simulink model "HDVSim_Dual_Fuel_Hybrid_Truck"  (R2018b)
settings: Solver=ode3  StartTime=0.0  StopTime=inf  FixedStep=sample_time  MaxStep=0.1  RelTol=1e-3  EnableMultiTasking=on
model workspace (MAT data in the model file):
  Bat.Useable_capacity = 30.52398723
  Bat.Useable_range = 0.302889592
  Bat.Type = 2
  Bat.SOC_start = 1
  Bat.Voltage = 800
  Bat.Charge_cycles = 14203.5582315
  Bat.Efficiency_power_electronics = 0.95
  Electric_Truck = 0
  Fueltype = 11
  Hybrid_Truck = 1
  IZ12 = 3600
  SOC_T_EM_completely_available = 0.089152566
  SOC_addition = 0.262901104
  SOC_target = 0
  Sailing_without_drag_torque = 1
  TCO = TCO
  TCO.Ratio_Trailer_Truck = [1 1]
  TCO.Price_increase_repurchase = [3.5 3.5]
  TCO.Daily_working_time = 8
  TCO.Other_works_day = 0.5
  TCO.Gross_hourly_wage_driver = 13
  TCO.Operating_days_year = 240
  TCO.Annual_gross_wage_driver = 24960
  TCO.Personnel_factor = 1.3
  TCO.Annual_gross_wage_truck = 32448
  TCO.Social_costs_percent = 25.75
  TCO.Social_costs_EUR = 8355
  TCO.Back_up_driver = 0
  TCO.Fees_day = 12
  TCO.Fees_year = 2880
  TCO.Driver_costs_other = 0
  TCO.Driving_personnel_costs_total = 43683
  TCO.Diesel_price = 0.95
  TCO.Diesel_price_external = 1
  TCO.Adblue_price = 0.68
  TCO.CNG_price = 0.88
  TCO.LNG_price = 0.81
  TCO.Electricity_price = 0.12
  TCO.Hydrogen_price = 9
  TCO.Interest_current_asset = 8.4
  TCO.Interest_fixed_asset = 8.4
  TCO.Administrative_costs = 10.7
  TCO.Driving_distance = 0
  TCO.Ratio_toll_route = 75
  TCO.Loading_time_combination = 0.25
  TCO.Unloading_time_combination = 0.25
  TCO.Ratio_empty_trips = 0
  TCO.Operating_life = [6 12]
  TCO.Tire_mileage = [140000 170000]
  TCO.Ratio_inhouse_tanking_diesel = 75
  TCO.Lubricant_consumption = 1
  TCO.Adblue_consumption = 4
  TCO.Afa_time_dependent = [100 100]
  TCO.Afa_power_dependent = [0 0]
  TCO.Current_asset = [6000 1400]
  TCO.Insurance_vehicle = [0 0]
  TCO.Insurance_transport = 1000
  TCO.Communication = 600
  TCO.Repair_maintenance_care = [0.13 0.025]
  TCO.Current_assets_interest_bearing = 622
  TCO.Results = table
  TCO.Results.data = {{[]; []; []; []; []; []; []; []; []; []; []; []; []; []; []; []; []; []; []; []; []; []; []}, {[]; []; []; []; []; []; []; []; []; []; []; []; []; []; []; []; []; []; []; []; []; []; []}, {[]; []; []; []; []; []; []; []; []; []; []; []; []; []; []; []; []; []; []; []; []; []; []}, {'#cccccc'; '#9DFF00'; '#CEFF00'; '#FFFF00'; '#FFDF00'; '#FFB900'; '#FF9200'; '#FF5D00'; '#FF7F7F'; '#FF2900'; '#cccccc'; '#00FF85'; '#00FFC6'; '#00FFF2'; '#00FFFF'; '#00DBFF'; '#00B3FF'; '#0088FF'; '#cccccc'; '#B100FF'; '#FF00FF'; '#FF00C0'; '#FF0070'}, [0; 1; 1; 1; 1; 1; 1; 0; 1; 0; 0; 1; 1; 1; 1; 1; 1; 0; 0; 0; 1; 1; 0]}
  TCO.Results.ndims = 2
  TCO.Results.nrows = 23
  TCO.Results.rownames = {'Time_dependent_vehicle_costs'; 'Amortisation_time_dependent'; 'Current_assets_interest_bearing'; 'Fixed_assets_interest_bearing'; 'Taxes'; 'Insurance'; 'Communication'; 'Sum_vehicle_costs'; 'Driving_personnel_costs_total'; 'Sum_fix_costs'; 'Performance_related_vehicle_costs'; 'Amortisation_performance_related'; 'Fuel_costs'; 'Adblue_costs'; 'Repair_costs'; 'Lubricant_costs'; 'Tire_costs'; 'Sum_variable_costs'; 'Sum_costs'; 'Sum_fix_variable_costs'; 'Overhead_costs'; 'Toll_costs'; 'Total_costs'}
  TCO.Results.nvars = 5
  TCO.Results.varnames = {'Euro_Year', 'Euro_km', 'Percent', 'Cellcolor', 'Diagramm'}
  TCO.Results.props.CustomProps = struct()
  TCO.Results.props.VariableCustomProps = struct()
  TCO.Results.props.versionSavedFrom = 3
  TCO.Results.props.minCompatibleVersion = 1
  TCO.Results.props.incompatibilityMsg = ''
  TCO.Results.props.VersionSavedFrom = 3
  TCO.Results.props.Description = ''
  TCO.Results.props.DimensionNames = {'Row', 'Variables'}
  TCO.Results.props.UserData = []
  TCO.Results.props.VariableDescriptions = {}
  TCO.Results.props.VariableUnits = {}
  TCO.Results.props.VariableContinuity = {}
  TCO_Trailer = 1
  T_distance_LPS_down = 500
  T_distance_LPS_up = 434.9496342
  VSim.Display = 3
  VSim.Opt = 0
  Vehicle = 'LNGDieselHybrid'
  WPT.Voltage = 0
  WPT.P_max = 200
  WPT.expansion = 0.3
  WPT.eta = 0.92
  WPT.SOC_target = 0.8
  WPT.SOC_electric_only = 0.3
  acquisitionCosts = acquisitionCosts
  acquisitionCosts.KA_ZM = 141266.812415
  acquisitionCosts.KG = 5816.60979338
  acquisitionCosts.Getr_m = 249.375588545
  acquisitionCosts.KMot = 21229.1233715
  acquisitionCosts.Motor_Mmax = 1810.391452
  acquisitionCosts.Motor_m = 882.849968657
  acquisitionCosts.KH = 16865.1016034
  acquisitionCosts.Hybrid = 1
  acquisitionCosts.Bat = 14389.2541556
  acquisitionCosts.Bat_type = 2
  acquisitionCosts.Bat_m = 500.750076074
  acquisitionCosts.Bat_kWh = 80.6207622479
  acquisitionCosts.Ratio_BEV2PHEV = 1
  acquisitionCosts.EM = 1329.27467614
  acquisitionCosts.EM_Type = 1
  acquisitionCosts.EM_P_max = 103.365060353
  acquisitionCosts.LE = 465.142771589
  acquisitionCosts.FC = 0
  acquisitionCosts.P_FC = 0
  acquisitionCosts.KA = 6181
  acquisitionCosts.v_diesel = 300
  acquisitionCosts.v_cng = 0
  acquisitionCosts.v_lng = 300
  acquisitionCosts.m_h2 = 0
  acquisitionCosts.KT = 4182.16
  acquisitionCosts.KTD = 292.81
  acquisitionCosts.KTCNG = 0
  acquisitionCosts.KTLNG = 3889.35
  acquisitionCosts.KTFC = 0
  addition_for_critical_slope = 0.030662181
  ambient.gravity = 9.80665
  ambient.air_density = 1.1883
  ambient.friction_coeff = 0.8
  auxiliary_consumers.onBattery = 0
  auxiliary_consumers.power = 3500
  critical_altitude_difference = 39.0505026
  cycle.distance = [0 1 2 3 4 5 6 7 8 9 10 11 ... (3001 elements, 3001x1)]
  cycle.speed = [0 24.16666667 24.16666667 24.16666667 24.16666667 24.16666667 24.16666667 24.16666667 24.16666667 24.16666667 24.16666667 24.16666667 ... (3001 elements, 3001x1)]
  cycle.slope = [0.0078 0.0078 0.0078 0.0078 0.0078 0.00779483187921 0.00777194955728 0.00778374504429 0.00779088449437 0.00779545771038 0.007798464127 0.00780054656295 ... (3001 elements, 3001x1)]
  cycle.stop_time = [5 0 0 0 0 0 0 0 0 0 0 0 ... (3001 elements, 3001x1)]
  cycle.altitude = [0 0 0 0 0 0 0 0 0 0 0 0 ... (3001 elements, 3001x1)]
  cycle.stop_end = 0
  cycle.stop_start = 5
  cycle.speed_init = 0
  cycle.delta12 = [0 0 0 0 0 0 0 0 0 0 0 0 ... (3001 elements, 1x3001)]
  cycle.delta23 = [0 0 0 0 0 0 0 0 0 0 0 0 ... (3001 elements, 1x3001)]
  dcycle = 5
  distance_1_PPC = 130
  distance_2_PPC = 290
  distance_PPC_altitude_difference = 4273.353363
  driver.controller_proportional_gain = 230000
  driver.controller_integral_gain = 3000
  driver.slew_rate_throttle_in = 2
  driver.slew_rate_throttle_out = -2
  driver.slew_rate_brake_in = 2
  driver.slew_rate_brake_out = -2
  em.P_max = 103.365060353
  em.M_max = 658.1057783
  em.n_eck = 1499.855571
  em.n_max = 2000
  em.shift_parameter.n_pref = 1409.86423674
  em.shift_parameter.n2 = 314.96966991
  em.shift_parameter.n6 = 1600
  em.shift_parameter.M_max = 658.1057783
  em.fuel.co2_per_kwh = 504
  em.speed = [0 10 20 30 40 50 60 70 80 90 100 110 120 130 140 150 160 170 180 190 200 210 220 230 240 250 260 270 280 290 300 310 320 330 340 350 360 370 380 390 400 410 420 430 440 450 460 470 480 490 500 510 520 530 540 550 560 570 580 590 600 610 620 630 640 650 660 670 680 690 700 710 720 730 740 750 760 770 780 790 800 810 820 830 840 850 860 870 880 890 900 910 920 930 940 950 960 970 980 990 1000 1010 1020 1030 1040 1050 1060 1070 1080 1090 1100 1110 1120 1130 1140 1150 1160 1170 1180 1190 1200 1210 1220 1230 1240 1250 1260 1270 1280 1290 1300 1310 1320 1330 1340 1350 1360 1370 1380 1390 1400 1410 1420 1430 1440 1450 1460 1470 1480 1490 1500 1510 1520 1530 1540 1550 1560 1570 1580 1590 1600 1610 1620 1630 1640 1650 1660 1670 1680 1690 1700 1710 1720 1730 1740 1750 1760 1770 1780 1790 1800 1810 1820 1830 1840 1850 1860 1870 1880 1890 1900 1910 1920 1930 1940 1950 1960 1970 1980 1990 2000]
  em.trq = [658.1057783 658.1057783 658.1057783 658.1057783 658.1057783 658.1057783 658.1057783 658.1057783 658.1057783 658.1057783 658.1057783 658.1057783 ... (201 elements, 1x201)]
  em.Type = 1
  em.efficiency.characteristic_map = [0.001 0.001 0.001 0.001 0.001 0.001 0.001 0.001 0.001 0.001 0.001 0.001 ... (20301 elements, 101x201)]
  em.efficiency.speed = [0 10 20 30 40 50 60 70 80 90 100 110 120 130 140 150 160 170 180 190 200 210 220 230 240 250 260 270 280 290 300 310 320 330 340 350 360 370 380 390 400 410 420 430 440 450 460 470 480 490 500 510 520 530 540 550 560 570 580 590 600 610 620 630 640 650 660 670 680 690 700 710 720 730 740 750 760 770 780 790 800 810 820 830 840 850 860 870 880 890 900 910 920 930 940 950 960 970 980 990 1000 1010 1020 1030 1040 1050 1060 1070 1080 1090 1100 1110 1120 1130 1140 1150 1160 1170 1180 1190 1200 1210 1220 1230 1240 1250 1260 1270 1280 1290 1300 1310 1320 1330 1340 1350 1360 1370 1380 1390 1400 1410 1420 1430 1440 1450 1460 1470 1480 1490 1500 1510 1520 1530 1540 1550 1560 1570 1580 1590 1600 1610 1620 1630 1640 1650 1660 1670 1680 1690 1700 1710 1720 1730 1740 1750 1760 1770 1780 1790 1800 1810 1820 1830 1840 1850 1860 1870 1880 1890 1900 1910 1920 1930 1940 1950 1960 1970 1980 1990 2000]
  em.efficiency.torque = [0 6.581057783 13.162115566 19.743173349 26.324231132 32.905288915 39.486346698 46.067404481 52.648462264 59.229520047 65.81057783 72.391635613 78.972693396 85.553751179 92.134808962 98.715866745 105.296924528 111.877982311 118.459040094 125.040097877 131.62115566 138.202213443 144.783271226 151.364329009 157.945386792 164.526444575 171.107502358 177.688560141 184.269617924 190.850675707 197.43173349 204.012791273 210.593849056 217.174906839 223.755964622 230.337022405 236.918080188 243.499137971 250.080195754 256.661253537 263.24231132 269.823369103 276.404426886 282.985484669 289.566542452 296.147600235 302.728658018 309.309715801 315.890773584 322.471831367 329.05288915 335.633946933 342.215004716 348.796062499 355.377120282 361.958178065 368.539235848 375.120293631 381.701351414 388.282409197 394.86346698 401.444524763 408.025582546 414.606640329 421.187698112 427.768755895 434.349813678 440.930871461 447.511929244 454.092987027 460.67404481 467.255102593 473.836160376 480.417218159 486.998275942 493.579333725 500.160391508 506.741449291 513.322507074 519.903564857 526.48462264 533.065680423 539.646738206 546.227795989 552.808853772 559.389911555 565.970969338 572.552027121 579.133084904 585.714142687 592.29520047 598.876258253 605.457316036 612.038373819 618.619431602 625.200489385 631.781547168 638.362604951 644.943662734 651.524720517 658.1057783]
  engine.bsfc.be = [0.158698130116 0.167286670662 0.175843316834 0.184367095709 0.192856917562 0.201311525468 0.209729386107 0.218108446837 0.226445614582 0.234735823164 0.242971531819 0.251147744004 ... (38000 elements, 190x200)]
  engine.bsfc.trqorig = [0 11.9341563786 23.8683127572 35.8024691358 47.7366255144 59.670781893 71.6049382716 83.5390946502 95.4732510288 107.407407407 119.341563786 131.275720165 ... (190 elements, 190x1)]
  engine.bsfc.speed = [563.093340492 570.821185914 578.549031336 586.276876758 594.00472218 601.732567602 609.460413023 617.188258445 624.916103867 632.643949289 640.371794711 648.099640133 ... (200 elements, 1x200)]
  engine.bsfc.M_be_min_orig = [1193.41563786 1205.34979424 1217.28395062 1229.218107 1241.15226337 1253.08641975 1253.08641975 1265.02057613 1276.95473251 1288.88888889 1300.82304527 1312.75720165 ... (200 elements, 1x200)]
  engine.bsfc.trq = [0 9.6798811356 19.3597622712 29.0396434068 38.7195245424 48.399405678 58.0792868136 67.7591679492 77.4390490848 87.1189302204 96.798811356 106.478692492 ... (190 elements, 190x1)]
  engine.bsfc.M_be_min = [967.98811356 977.667994695 987.347875831 997.027756966 1006.7076381 1016.38751924 1016.38751924 1026.06740037 1035.74728151 1045.42716264 1055.10704378 1064.78692492 ... (200 elements, 1x200)]
  engine.full_load.trqorig = [1193.41563786 1205.34979424 1217.28395062 1229.218107 1241.15226337 1253.08641975 1253.08641975 1265.02057613 1276.95473251 1288.88888889 1300.82304527 1312.75720165 ... (200 elements, 1x200)]
  engine.full_load.speed = [563.093340492 570.821185914 578.549031336 586.276876758 594.00472218 601.732567602 609.460413023 617.188258445 624.916103867 632.643949289 640.371794711 648.099640133 ... (200 elements, 1x200)]
  engine.full_load.trq = [967.98811356 977.667994695 987.347875831 997.027756966 1006.7076381 1016.38751924 1016.38751924 1026.06740037 1035.74728151 1045.42716264 1055.10704378 1064.78692492 ... (200 elements, 1x200)]
  engine.full_load.power = [57.0793519229 58.4413311666 59.8189774543 61.2122907861 62.6212711619 64.0459185818 64.8684383943 66.3165863802 67.7804014102 69.2598834842 70.7550326023 72.2658487645 ... (200 elements, 1x200)]
  engine.number = 2
  engine.M_max_original = 2232
  engine.M_max = 1810.391452
  engine.scale_factor = 0.811107281362
  engine.speed_min = 800
  engine.speed_max = 2100
  engine.idle_fuel_consumption = 1
  engine.drag_torque.trq = [-97.3328737634 -210.887893154]
  engine.drag_torque.speed = [600 2190]
  engine.shift_parameter.n_lo = 1020.247354
  engine.shift_parameter.n_pref = 1265.144022
  engine.shift_parameter.n1 = 600
  engine.shift_parameter.n2 = 800
  engine.shift_parameter.n3 = 1142.695688
  engine.shift_parameter.n4 = 800
  engine.shift_parameter.n5 = 1265.144022
  engine.shift_parameter.n6 = 2100
  engine.shift_parameter.M_max = 1810.13777236
  engine.fuel.density_diesel = 0.83
  engine.fuel.co2_per_litre_diesel = 2.62
  engine.fuel.co2_per_kg_gas = 2.75
  engine.fuel.heat_of_combustion = 49587.8
  engine.fuel.Gasart = 'LNG'
  final_drive.ratio = 2.860669464
  final_drive.trq_eff = 0.98
  ifElectric = 0
  ifOptimized = 1
  look_ahead_PPC = 920
  max_distance = 3000
  name = 'HDVSim_Dual_Fuel_Hybrid_Truck'
  preditiveCruiseControl = 1
  sample_time = 0.1
  tank.v_diesel = 300
  tank.v_cng = 0
  tank.v_lng = 300
  tank.m_h2 = 0
  tires.radius = 0.4465
  tires.roll_drag_coeff.total = 0.0043
  transmission.init_gear = 1
  transmission.shift_time = 1
  transmission.ratios = [17.07936487 12.4603549715 9.09052808455 6.63205029428 4.83845280459 3.52992279966 2.5752767413 1.8788088779 1.37069649372 1]
  transmission.trq_eff = [0.96 0.96 0.96 0.96 0.98 0.97 0.97 0.97 0.97 0.99]
  transmission.lamda = [1.29195493417 1.12426696173 1.06303842304 1.03085329001 1.02049678901 1.01315441026 1.01055516169 1.00846776899 1.00728485922 1.0060193999]
  transmission.z = 10
  v_PPC_delta = 2.77123754361
  v_max_electrical_drive_only = 9.22694367778
  vehicle.long_truck = 0
  vehicle.payload = 19300
  vehicle.frontal_area = 10.2
  vehicle.air_drag_coeff = 0.53
  vehicle.Fx_max = 90221.18
  vehicle.F_brake_max = 309890.14
  vehicle.mass = 13313.038289
  vehicleProperties = vehicleProperties
  vehicleProperties.CO2_EM_Range = 100
  vehicleProperties.a_0_80_Range = 54
  vehicleProperties.BOK_ak = 2.55
  vehicleProperties.BOK_Range = 4.65
  vehicleProperties.V_Rel_ak = 0.55
  vehicleProperties.V_Rel_Range = 0.35
  vehicleProperties.VWF_ak = 0.9
  vehicleProperties.VWF_Range = 7.2
  weights = weights
  weights.m_Engine = 882.849968657
  weights.m_Gearbox = 249.375588545
  weights.m_Retarder = 82
  weights.m_tank_system = 278.209286611
  weights.m_Fuel = 417
  weights.m_Exhaust = 203.4
  weights.m_Battery = 500.750076074
  weights.m_EM = 51.6825301765
  weights.m_PwrElectr = 9.57083892158
  weights.m_Charger = 15
  weights.m_Trailer = 5400
  weights.m_Total = 7913.03828899
  weights.m_Base = 5223.2
  weights.Hybrid = 1
  weights.max_Payload = 27686.961711
  weights.m_Max = 41000
  x = [17.07936487 6 0 0 2.860669464 1810.391452 1020.247354 1265.144022 9.976455157 83 4 20 658.1057783 1499.855571 30.52398723 0 0.089152566 33.21699724 434.9496342 500 0.030662181 4273.353363 39.0505026 0.262901104 0.302889592 2 1]
values from neighbouring files (symbols this model uses):
  transmission = Transmission_gearing(1, 1, false, false, final_drive.ratio)    [Parameterizing.m]
undefined symbols (not defined in the file or in its folder): Hybrid_LKW, Ion, Lithium
libraries: simulink x22, powerlib x2, electricdrivelib x1
(part 1 of 3)
settings Model: Creator=Alexander Suessmann  LastModifiedBy=ga73rep
settings DataIOCC: SaveFormat=Array  SignalLoggingSaveFormat=ModelDataLogs  SaveOutput=off  SignalLogging=off  DSMLogging=off  SignalLoggingName=datalog
settings OptimizationCC: ExpressionDepthLimit=2147483647  InitFltsAndDblsToZero=on  LifeSpan=inf
settings DebuggingCC: UnderspecifiedInitializationDetection=Classic  MergeDetectMultiDrivingBlocksExec=none  SolverPrmCheckMsg=warning  MultiTaskDSMMsg=warning  MultiTaskCondExecSysMsg=none  FcnCallInpInsideContextMsg=warning  AllowSymbolicDim=off  StateNameClashWarn=warning  LibraryContextMissingDiagnostic=none  SFUnexpectedBacktrackingDiag=warning  SFNoUnconditionalDefaultTransitionDiag=warning  SFExecutionAtInitializationDiag=none
settings HardwareCC: ProdBitPerPointer=32  ProdBitPerSizeT=32  ProdBitPerPtrDiffT=32  ProdLargestAtomicFloat=None  ProdIntDivRoundTo=Undefined  ProdEndianess=Unspecified  ProdWordSize=32  ProdHWDeviceType=32-bit Generic
settings ModelReferenceCC: PropagateSignalLabelsOutOfModel=off
settings SFSimCC: SimUseLocalCustomCode=off
settings RTWCC: RTWUseLocalCustomCode=off
settings CodeAppCC: StateflowObjectComments=on
settings GRTTargetCC: TargetLangStandard=C89/C90 (ANSI)  GeneratePreprocessorConditionals=Disable all  CombineOutputUpdateFcns=off  GRTInterface=on
settings ConfigComp: CovMetricSettings=dw  CovHtmlReporting=on  CovSaveCumulativeToWorkspaceVar=on  CovSaveSingleToWorkspaceVar=on  CovExternalEMLEnable=off
settings SimscapeCC: SimscapeNormalizeSystem=off

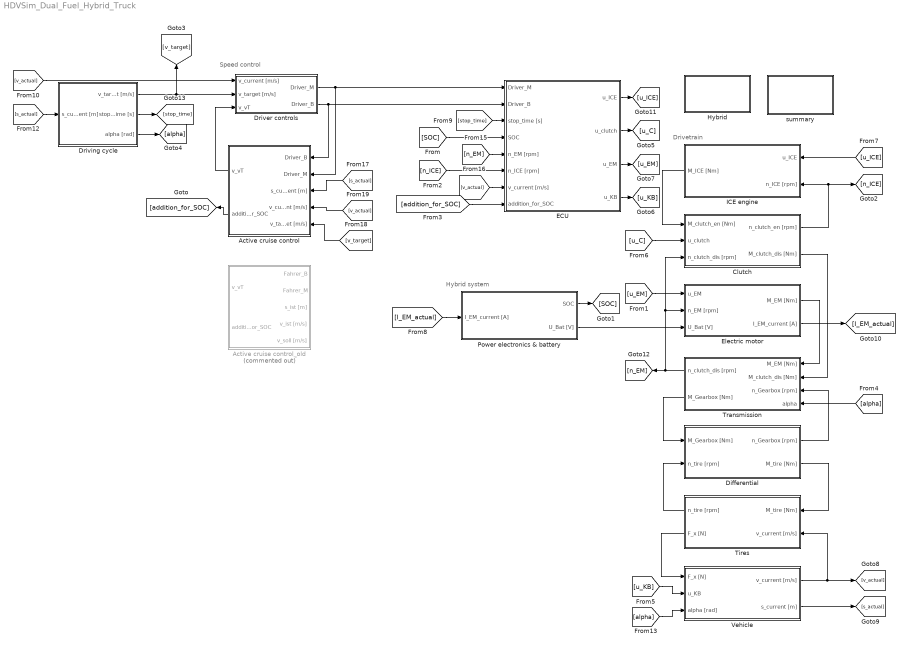
== system HDVSim_Dual_Fuel_Hybrid_Truck ==
  note: Hybrid system
  note: Drivetrain
  note: Speed control
  Active cruise control : Subsystem
  Active cruise control_old : Subsystem  Commented=on
  Clutch : Subsystem
  Differential : Subsystem
  Driver controls : Subsystem
  Driving cycle : Subsystem
  ECU : Subsystem
  Electric motor : Subsystem
  Hybrid : Subsystem
  ICE engine : Subsystem
  Power electronics & battery : Subsystem
  Tires : Subsystem
  Transmission : Subsystem
  Vehicle : Subsystem
  summary : Subsystem
  wires:
  ICE engine/1(M_ICE [Nm]) -> Clutch/1(M_clutch_en [Nm])
  Transmission/1(n_clutch_dis [rpm]) -> Clutch/3(n_clutch_dis [rpm]), Electric motor/2(n_EM [rpm]), [n_EM]
  Transmission/2(M_Gearbox [Nm]) -> Differential/1(M_Gearbox [Nm])
  Tires/1(n_tire [rpm]) -> Differential/2(n_tire [rpm])
  Clutch/1(n_clutch_en [rpm]) -> ICE engine/2(n_ICE [rpm]), [n_ICE]
  Clutch/2(M_clutch_dis [Nm]) -> Transmission/2(M_clutch_dis [Nm])
  Differential/1(n_Gearbox [rpm]) -> Transmission/3(n_Gearbox [rpm])
  Differential/2(M_tire [Nm]) -> Tires/1(M_tire [Nm])
  Tires/2(F_x [N]) -> Vehicle/1(F_x [N])
  Electric motor/1(M_EM [Nm]) -> Transmission/1(M_EM [Nm])
  Power electronics & battery/2(U_Bat [V]) -> Electric motor/3(U_Bat [V])
  Driving cycle/1(v_target [m/s]) -> [v_target], Driver controls/2(v_target [m/s])
  Active cruise control/1(v_vT) -> Driver controls/3(v_vT)
  Vehicle/1(v_current [m/s]) -> [v_actual], Tires/2(v_current [m/s])
  Active cruise control/2(addition_for_SOC) -> [addition_for_SOC]
  Power electronics & battery/1(SOC) -> [SOC]
  [v_actual] -> Driver controls/1(v_current [m/s])
  Driver controls/1(Driver_M) -> Active cruise control/2(Driver_M), ECU/1(Driver_M)
  Driver controls/2(Driver_B) -> Active cruise control/1(Driver_B), ECU/2(Driver_B)
  [s_actual] -> Active cruise control/3(s_current [m])
  [v_actual] -> Active cruise control/4(v_current [m/s])
  [v_target] -> Active cruise control/5(v_target [m/s])
  [addition_for_SOC] -> ECU/8(addition_for_SOC)
  [n_ICE] -> ECU/6(n_ICE [rpm])
  [SOC] -> ECU/4(SOC)
  [n_EM] -> ECU/5(n_EM [rpm])
  [v_actual] -> ECU/7(v_current [m/s])
  Driving cycle/3(alpha [rad]) -> [alpha]
  [s_actual] -> Driving cycle/1(s_current [m])
  ECU/1(u_ICE) -> [u_ICE]
  ECU/2(u_clutch) -> [u_C]
  ECU/3(u_EM) -> [u_EM]
  ECU/4(u_KB) -> [u_KB]
  [u_C] -> Clutch/2(u_clutch)
  [u_EM] -> Electric motor/1(u_EM)
  [u_ICE] -> ICE engine/1(u_ICE)
  Electric motor/2(I_EM_current [A]) -> [I_EM_actual]
  [alpha] -> Transmission/4(alpha)
  Vehicle/2(s_current [m]) -> [s_actual]
  [u_KB] -> Vehicle/2(u_KB)
  [alpha] -> Vehicle/3(alpha [rad])
  [I_EM_actual] -> Power electronics & battery/1(I_EM_current [A])
  Driving cycle/2(stop_time [s]) -> [stop_time]
  [stop_time] -> ECU/3(stop_time [s])

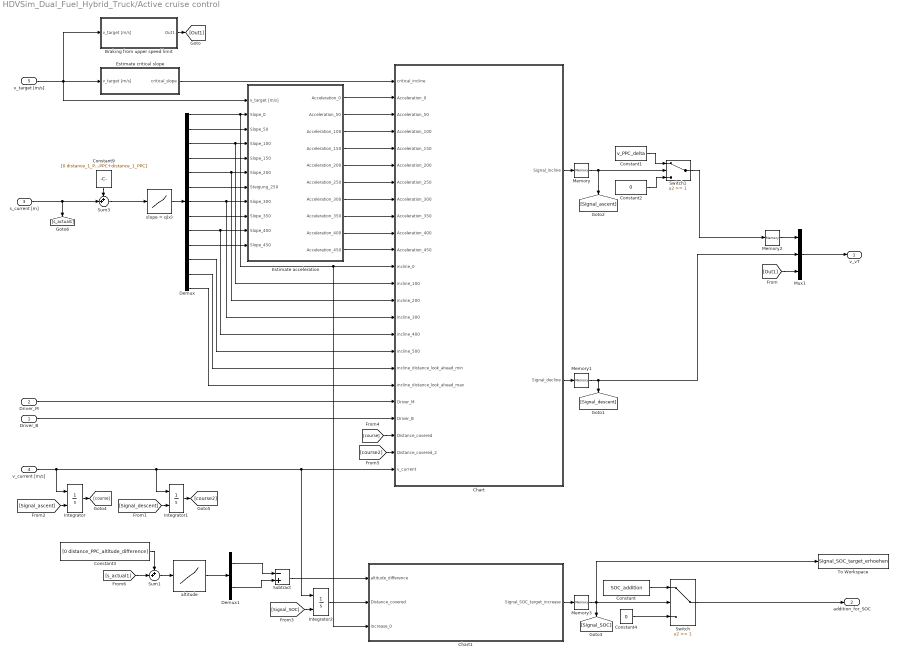
== system HDVSim_Dual_Fuel_Hybrid_Truck/Active cruise control ==
  Driver_B : Inport
  Driver_M : Inport  Port=2
  s_current [m] : Inport  Port=3
  v_current [m/s] : Inport  Port=4
  v_target [m/s] : Inport  Port=5
  Braking from upper speed limit : Subsystem
  Chart : Stateflow chart  TreatAsAtomicUnit=on
  Chart1 : Stateflow chart  TreatAsAtomicUnit=on
  Constant : Constant  Value=SOC_addition
  Constant1 : Constant  Value=v_PPC_delta
  Constant2 : Constant  Value=0
  Constant3 : Constant  Value=[0 distance_PPC_altitude_difference]
  Constant4 : Constant  Value=0
  Constant9 : Constant  Value=[0 distance_1_PPC/5 2*distance_1_PPC/5 3*distance_1_PPC/5 4*distance_1_PPC/5 distance_1_PPC 6*distance_1_PPC/5 7*distance_1_PPC/5 8*distance_1_PPC/5 9*distance_1_PPC/5 10*distance_1_PPC/5 look_ahead_PPC look_ahead_PPC+distance_1_PPC]
  Demux : Demux  Outputs=13
  Demux1 : Demux  Outputs=2
  Estimate acceleration : Subsystem
  Estimate critical slope : Subsystem
  Integrator : Integrator  ExternalReset=rising
  Integrator1 : Integrator  ExternalReset=rising
  Integrator2 : Integrator  ExternalReset=rising
  Memory{,1..3} (4 alike) : Memory
  Mux1 : Mux  Inputs=3
  Subtract : Sum  Inputs=-+
  Sum1 : Sum  Inputs=++|
  Sum3 : Sum  Inputs=++|
  Switch : Switch  Threshold=1
  Switch1 : Switch  Threshold=1
  To Workspace : ToWorkspace  VariableName=Signal_SOC_target_erhoehen  SaveFormat=Structure With Time  SampleTime=-1
  altitude : Lookup_n-D  NumberOfTableDimensions=1  BreakpointsForDimension1=cycle.distance  Table=cycle.altitude  InterpMethod=Flat  RndMeth=Simplest  InputSameDT=on
  slope = q(x) : Lookup  InputValues=cycle.distance  Table=cycle.slope  LookUpMeth=Interpolation-Use End Values
  v_vT : Outport
  addition_for_SOC : Outport  Port=2
  wires:
  slope = q(x)/1 -> Demux/1
  Demux/1 -> Chart1/3(increase_0), Chart/12(incline_0), Estimate acceleration/2(Slope_0)
  Chart/1(Signal_incline) -> Memory/1
  v_current [m/s]/1 -> Integrator/1, Integrator1/1, Integrator2/1, Chart/24(v_current)
  Memory/1 -> [Signal_ascent], Switch1/2
  Mux1/1 -> v_vT/1
  Constant9/1 -> Sum3/1
  Sum3/1 -> slope = q(x)/1
  Estimate acceleration/1(Acceleration_0) -> Chart/2(Acceleration_0)
  Estimate acceleration/2(Acceleration_50) -> Chart/3(Acceleration_50)
  Estimate acceleration/3(Acceleration_100) -> Chart/4(Acceleration_100)
  Estimate acceleration/4(Acceleration_150) -> Chart/5(Acceleration_150)
  Estimate acceleration/5(Acceleration_200) -> Chart/6(Acceleration_200)
  Estimate acceleration/6(Acceleration_250) -> Chart/7(Acceleration_250)
  Estimate acceleration/7(Acceleration_300) -> Chart/8(Acceleration_300)
  Estimate acceleration/8(Acceleration_350) -> Chart/9(Acceleration_350)
  Chart/2(Signal_decline) -> Memory1/1
  Memory1/1 -> Mux1/2, [Signal_descent]
  Driver_B/1 -> Chart/21(Driver_B)
  Estimate acceleration/9(Acceleration_400) -> Chart/10(Acceleration_400)
  Estimate acceleration/10(Acceleration_450) -> Chart/11(Acceleration_450)
  Driver_M/1 -> Chart/20(Driver_M)
  Demux/2 -> Estimate acceleration/3(Slope_50)
  Demux/3 -> Chart/13(incline_100), Estimate acceleration/4(Slope_100)
  Demux/4 -> Estimate acceleration/5(Slope_150)
  Demux/5 -> Chart/14(incline_200), Estimate acceleration/6(Slope_200)
  Demux/6 -> Estimate acceleration/7("Steigung_250 ")
  Demux/7 -> Chart/15(incline_300), Estimate acceleration/8(Slope_300)
  Demux/8 -> Estimate acceleration/9(Slope_350)
  Demux/9 -> Chart/16(incline_400), Estimate acceleration/10(Slope_400)
  Demux/10 -> Estimate acceleration/11(Slope_450)
  Demux/12 -> Chart/18(incline_distance_look_ahead_min)
  Demux/13 -> Chart/19(incline_distance_look_ahead_max)
  v_target [m/s]/1 -> Estimate critical slope/1(v_target [m/s]), Braking from upper speed limit/1(v_target [m/s]), Estimate acceleration/1(v_target [m/s])
  Memory2/1 -> Mux1/1
  Constant1/1 -> Switch1/1
  Constant2/1 -> Switch1/3
  Demux/11 -> Chart/17(incline_500)
  Switch1/1 -> Memory2/1
  Constant3/1 -> Sum1/1
  s_current [m]/1 -> [s_actual1], Sum3/2
  Sum1/1 -> altitude/1
  altitude/1 -> Demux1/1
  Demux1/2 -> Subtract/2
  Demux1/1 -> Subtract/1
  Subtract/1 -> Chart1/1(altitude_difference)
  Chart1/1(Signal_SOC_target_increase) -> Memory3/1
  Integrator2/1 -> Chart1/2(Distance_covered)
  Constant/1 -> Switch/1
  Constant4/1 -> Switch/3
  Switch/1 -> addition_for_SOC/1
  Memory3/1 -> Switch/2, To Workspace/1, [Signal_SOC]
  [Signal_descent] -> Integrator1/2
  Integrator1/1 -> [course2]
  Integrator/1 -> [course]
  [Signal_ascent] -> Integrator/2
  [course] -> Chart/22(Distance_covered)
  [course2] -> Chart/23(Distance_covered_2)
  [Signal_SOC] -> Integrator2/2
  [s_actual1] -> Sum1/2
  Braking from upper speed limit/1(Out1) -> [Out1]
  [Out1] -> Mux1/3
  Estimate critical slope/1(critical_slope) -> Chart/1(critical_incline)

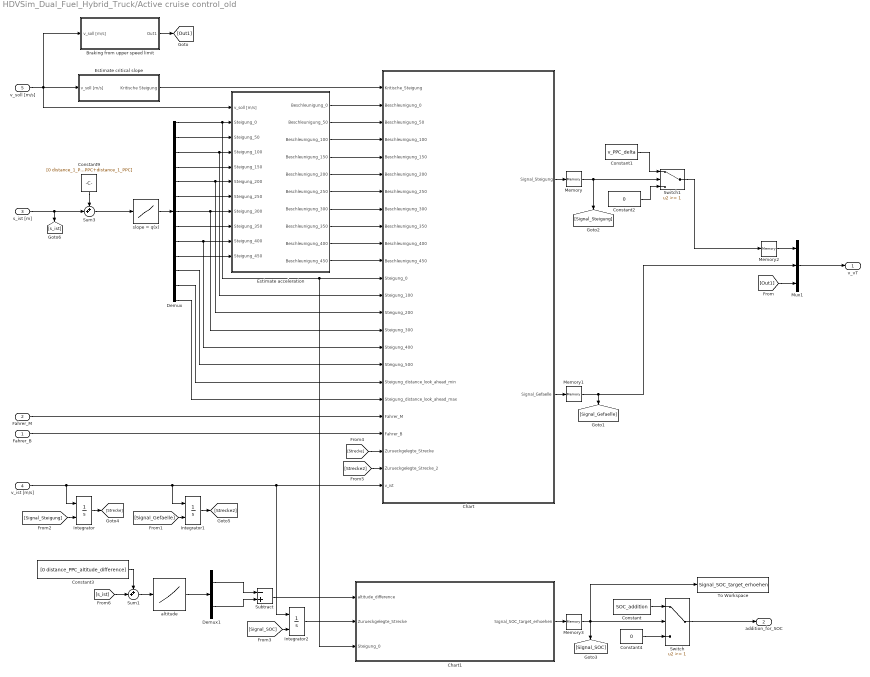
== system HDVSim_Dual_Fuel_Hybrid_Truck/Active cruise control_old ==
  Fahrer_B : Inport
  Fahrer_M : Inport  Port=2
  s_ist [m] : Inport  Port=3
  v_ist [m/s] : Inport  Port=4
  v_soll [m/s] : Inport  Port=5
  Braking from upper speed limit : Subsystem
  Chart : Stateflow chart  TreatAsAtomicUnit=on
  Chart1 : Stateflow chart  TreatAsAtomicUnit=on
  Constant : Constant  Value=SOC_addition
  Constant1 : Constant  Value=v_PPC_delta
  Constant2 : Constant  Value=0
  Constant3 : Constant  Value=[0 distance_PPC_altitude_difference]
  Constant4 : Constant  Value=0
  Constant9 : Constant  Value=[0 distance_1_PPC/5 2*distance_1_PPC/5 3*distance_1_PPC/5 4*distance_1_PPC/5 distance_1_PPC 6*distance_1_PPC/5 7*distance_1_PPC/5 8*distance_1_PPC/5 9*distance_1_PPC/5 10*distance_1_PPC/5 look_ahead_PPC look_ahead_PPC+distance_1_PPC]
  Demux : Demux  Outputs=13
  Demux1 : Demux  Outputs=2
  Estimate acceleration : Subsystem
  Estimate critical slope : Subsystem
  Integrator : Integrator  ExternalReset=rising
  Integrator1 : Integrator  ExternalReset=rising
  Integrator2 : Integrator  ExternalReset=rising
  Memory{,1..3} (4 alike) : Memory
  Mux1 : Mux  Inputs=3
  Subtract : Sum  Inputs=-+
  Sum1 : Sum  Inputs=++|
  Sum3 : Sum  Inputs=++|
  Switch : Switch  Threshold=1
  Switch1 : Switch  Threshold=1
  To Workspace : ToWorkspace  VariableName=Signal_SOC_target_erhoehen  SaveFormat=Structure With Time  SampleTime=-1
  altitude : Lookup_n-D  NumberOfTableDimensions=1  BreakpointsForDimension1=cycle.distance  Table=cycle.altitude  InterpMethod=Flat  RndMeth=Simplest  InputSameDT=on
  slope = q(x) : Lookup  InputValues=cycle.distance  Table=cycle.slope  LookUpMeth=Interpolation-Use End Values
  v_vT : Outport
  addition_for_SOC : Outport  Port=2
  wires:
  slope = q(x)/1 -> Demux/1
  Demux/1 -> Estimate acceleration/2(Steigung_0), Chart1/3(Steigung_0), Chart/12(Steigung_0)
  Estimate critical slope/1(Kritische Steigung) -> Chart/1(Kritische_Steigung)
  Chart/1(Signal_Steigung) -> Memory/1
  Memory/1 -> [Signal_Steigung], Switch1/2
  Mux1/1 -> v_vT/1
  Constant9/1 -> Sum3/1
  Sum3/1 -> slope = q(x)/1
  Estimate acceleration/1(Beschleunigung_0) -> Chart/2(Beschleunigung_0)
  Estimate acceleration/2(Beschleunigung_50) -> Chart/3(Beschleunigung_50)
  Estimate acceleration/3(Beschleunigung_100) -> Chart/4(Beschleunigung_100)
  Estimate acceleration/4(Beschleunigung_150) -> Chart/5(Beschleunigung_150)
  Estimate acceleration/5(Beschleunigung_200) -> Chart/6(Beschleunigung_200)
  Estimate acceleration/6(Beschleunigung_250) -> Chart/7(Beschleunigung_250)
  Estimate acceleration/7(Beschleunigung_300) -> Chart/8(Beschleunigung_300)
  Estimate acceleration/8(Beschleunigung_350) -> Chart/9(Beschleunigung_350)
  Chart/2(Signal_Gefaelle) -> Memory1/1
  Memory1/1 -> [Signal_Gefaelle], Mux1/2
  Fahrer_B/1 -> Chart/21(Fahrer_B)
  Estimate acceleration/9(Beschleunigung_400) -> Chart/10(Beschleunigung_400)
  Estimate acceleration/10(Beschleunigung_450) -> Chart/11(Beschleunigung_450)
  Fahrer_M/1 -> Chart/20(Fahrer_M)
  Demux/2 -> Estimate acceleration/3(Steigung_50)
  Demux/3 -> Chart/13(Steigung_100), Estimate acceleration/4(Steigung_100)
  Demux/4 -> Estimate acceleration/5(Steigung_150)
  Demux/5 -> Chart/14(Steigung_200), Estimate acceleration/6(Steigung_200)
  Demux/6 -> Estimate acceleration/7("Steigung_250 ")
  Demux/7 -> Chart/15(Steigung_300), Estimate acceleration/8(Steigung_300)
  Demux/8 -> Estimate acceleration/9(Steigung_350)
  Demux/9 -> Chart/16(Steigung_400), Estimate acceleration/10(Steigung_400)
  Demux/10 -> Estimate acceleration/11(Steigung_450)
  Demux/12 -> Chart/18(Steigung_distance_look_ahead_min)
  Demux/13 -> Chart/19(Steigung_distance_look_ahead_max)
  v_soll [m/s]/1 -> Braking from upper speed limit/1(v_soll [m/s]), Estimate acceleration/1(v_soll [m/s]), Estimate critical slope/1(v_soll [m/s])
  Memory2/1 -> Mux1/1
  Constant1/1 -> Switch1/1
  Constant2/1 -> Switch1/3
  Demux/11 -> Chart/17(Steigung_500)
  Switch1/1 -> Memory2/1
  Constant3/1 -> Sum1/1
  s_ist [m]/1 -> [s_ist], Sum3/2
  Sum1/1 -> altitude/1
  altitude/1 -> Demux1/1
  Demux1/2 -> Subtract/2
  Demux1/1 -> Subtract/1
  Subtract/1 -> Chart1/1(altitude_difference)
  Chart1/1(Signal_SOC_target_erhoehen) -> Memory3/1
  Integrator2/1 -> Chart1/2(Zurueckgelegte_Strecke)
  Constant/1 -> Switch/1
  Constant4/1 -> Switch/3
  Switch/1 -> addition_for_SOC/1
  Memory3/1 -> To Workspace/1, [Signal_SOC], Switch/2
  Braking from upper speed limit/1(Out1) -> [Out1]
  v_ist [m/s]/1 -> Integrator/1, Integrator1/1, Integrator2/1, Chart/24(v_ist)
  Integrator/1 -> [Strecke]
  Integrator1/1 -> [Strecke2]
  [Signal_Gefaelle] -> Integrator1/2
  [Signal_Steigung] -> Integrator/2
  [Strecke2] -> Chart/23(Zurueckgelegte_Strecke_2)
  [Strecke] -> Chart/22(Zurueckgelegte_Strecke)
  [s_ist] -> Sum1/2
  [Signal_SOC] -> Integrator2/2
  [Out1] -> Mux1/3

== system HDVSim_Dual_Fuel_Hybrid_Truck/Clutch ==
  note: Torque where clutch is disengaged
  note: Speed where clutch is engaged
  M_clutch_en [Nm] : Inport
  u_clutch : Inport  Port=2
  n_clutch_dis [rpm] : Inport  Port=3
  Compare To Zero : simulink/Logic and Bit Operations/Compare To Zero  relop===  OutDataTypeStr=boolean
  Constant : Constant  Value=0
  Idle engine speed : Constant  Value=engine.speed_min
  Logical Operator : Logic  AllPortsSameDT=off  OutDataTypeStr=boolean
  Lower engine speed : Saturate  UpperLimit=10000  LowerLimit=engine.speed_min  ZeroCross=off
  Null1 : Constant  Value=0
  Switch1 : Switch  Threshold=1
  Switch2 : Switch  Threshold=1
  Switch3 : Switch  Threshold=1
  n_clutch_en [rpm] : Outport
  M_clutch_dis [Nm] : Outport  Port=2
  wires:
  n_clutch_dis [rpm]/1 -> Lower engine speed/1
  Lower engine speed/1 -> Switch3/3
  Switch2/1 -> Switch1/3
  Null1/1 -> Switch2/1
  M_clutch_en [Nm]/1 -> Switch2/3
  [M_mot] -> Compare To Zero/1
  Compare To Zero/1 -> Logical Operator/1
  [ZKU] -> Logical Operator/2
  Logical Operator/1 -> Switch2/2
  Switch1/1 -> M_clutch_dis [Nm]/1
  Constant/1 -> Switch1/1
  Switch3/1 -> n_clutch_en [rpm]/1
  u_clutch/1 -> Switch1/2, Switch3/2
  Idle engine speed/1 -> Switch3/1

== system HDVSim_Dual_Fuel_Hybrid_Truck/Differential ==
  note: Effective wheel torque
  M_Gearbox [Nm] : Inport
  n_tire [rpm] : Inport  Port=2
  Differential efficiency : Constant  Value=final_drive.trq_eff
  Differential gear ratio : Constant  Value=final_drive.ratio
  M' = M*i*eta : Product  Inputs=***
  Product : Product  Inputs=/  RndMeth=Zero
  Switch : Switch  ZeroCross=off
  n' *i = n : Product  RndMeth=Zero
  n_Gearbox [rpm] : Outport
  M_tire [Nm] : Outport  Port=2
  tag scope: Eta_axle_drive=global
  wires:
  M_Gearbox [Nm]/1 -> M' = M*i*eta/1, Switch/2
  n_tire [rpm]/1 -> n' *i = n/2
  Differential gear ratio/1 -> n' *i = n/1, M' = M*i*eta/3
  n' *i = n/1 -> n_Gearbox [rpm]/1
  M' = M*i*eta/1 -> M_tire [Nm]/1
  Differential efficiency/1 -> Product/1, Switch/1
  Product/1 -> Switch/3
  Switch/1 -> [Eta_axle_drive], M' = M*i*eta/2

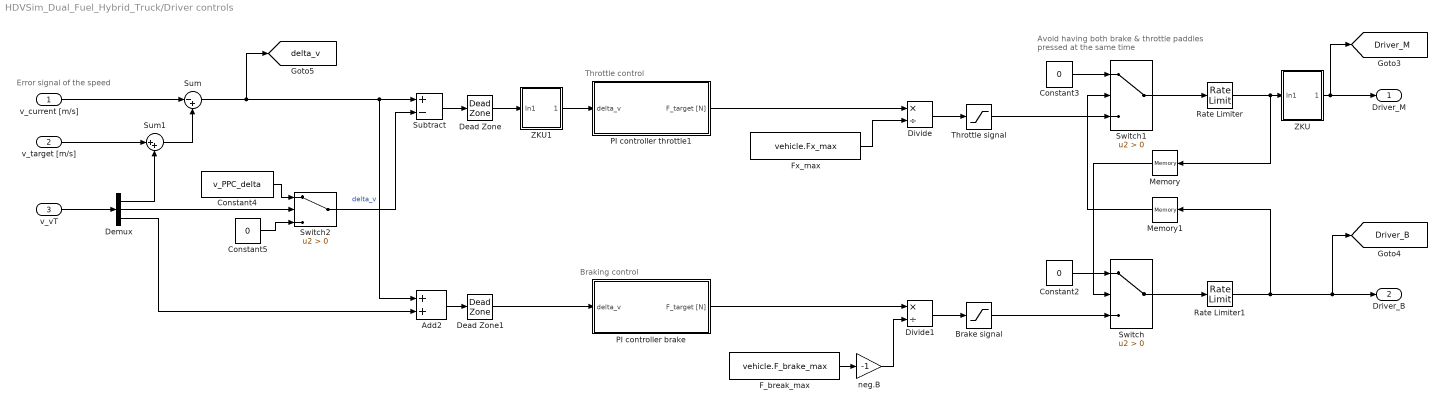
== system HDVSim_Dual_Fuel_Hybrid_Truck/Driver controls ==
  note: Error signal of the speed
  note: Throttle control
  note: Avoid having both brake & throttle
      | paddles pressed at the same time
  note: Braking control
  v_current [m/s] : Inport
  v_target [m/s] : Inport  Port=2
  v_vT : Inport  Port=3
  Add2 : Sum
  Brake signal : Saturate  UpperLimit=1  LowerLimit=0  ZeroCross=off
  Constant2 : Constant  Value=0
  Constant3 : Constant  Value=0
  Constant4 : Constant  Value=v_PPC_delta
  Constant5 : Constant  Value=0
  Dead Zone : DeadZone  LowerValue=-0.1/3.6  UpperValue=0.1/3.6  ZeroCross=off  SaturateOnIntegerOverflow=on
  Dead Zone1 : DeadZone  LowerValue=-0.1/3.6  UpperValue=0  ZeroCross=off  SaturateOnIntegerOverflow=on
  Demux : Demux  Outputs=3
  Divide : Product  Inputs=*/
  Divide1 : Product  Inputs=*/
  F_break_max : Constant  Value=vehicle.F_brake_max
  Fx_max : Constant  Value=vehicle.Fx_max
  Memory : Memory
  Memory1 : Memory
  PI controller brake : Subsystem
  PI controller throttle1 : Subsystem
  Rate Limiter : RateLimiter  RisingSlewLimit=driver.slew_rate_throttle_in  FallingSlewLimit=driver.slew_rate_throttle_out  SampleTimeMode=inherited
  Rate Limiter1 : RateLimiter  RisingSlewLimit=driver.slew_rate_brake_in*100  FallingSlewLimit=driver.slew_rate_brake_out*100  SampleTimeMode=inherited
  Subtract : Sum  Inputs=+-
  Sum : Sum  Inputs=|-+
  Sum1 : Sum  Inputs=|++
  Switch : Switch  Criteria=u2 > Threshold
  Switch1 : Switch  Criteria=u2 > Threshold
  Switch2 : Switch  Criteria=u2 > Threshold
  Throttle signal : Saturate  UpperLimit=1  LowerLimit=0  ZeroCross=off
  ZKU : Subsystem
  ZKU1 : Subsystem
  neg.B : Gain  Gain=-1
  Driver_M : Outport
  Driver_B : Outport  Port=2
  tag scope: Driver_B=global, Driver_M=global, delta_v=global
  wires:
  Sum1/1 -> Sum/2
  v_current [m/s]/1 -> Sum/1
  Fx_max/1 -> Divide/2
  neg.B/1 -> Divide1/2
  Sum/1 -> [delta_v], Add2/1, Subtract/1  "delta_v"
  Divide1/1 -> Brake signal/1
  Divide/1 -> Throttle signal/1
  F_break_max/1 -> neg.B/1
  Switch/1 -> Rate Limiter1/1
  Brake signal/1 -> Switch/3
  Constant2/1 -> Switch/1
  Switch1/1 -> Rate Limiter/1
  Throttle signal/1 -> Switch1/3
  Rate Limiter1/1 -> Memory1/1, [Driver_B], Driver_B/1
  Rate Limiter/1 -> ZKU/1(In1), Memory/1
  Constant3/1 -> Switch1/1
  PI controller throttle1/1(F_target [N]) -> Divide/1
  Dead Zone/1 -> ZKU1/1(In1)
  Dead Zone1/1 -> PI controller brake/1(delta_v)
  PI controller brake/1(F_target [N]) -> Divide1/1
  ZKU/1(Out1) -> [Driver_M], Driver_M/1
  ZKU1/1(Out1) -> PI controller throttle1/1(delta_v)
  Memory/1 -> Switch/2
  Memory1/1 -> Switch1/2
  v_vT/1 -> Demux/1
  Switch2/1 -> Subtract/2
  Demux/2 -> Switch2/2
  Constant4/1 -> Switch2/1
  Constant5/1 -> Switch2/3
  Subtract/1 -> Dead Zone/1
  Demux/1 -> Sum1/2
  v_target [m/s]/1 -> Sum1/1
  Demux/3 -> Add2/2
  Add2/1 -> Dead Zone1/1

== system HDVSim_Dual_Fuel_Hybrid_Truck/Driving cycle ==
  note: Lookup tables
  s_current [m] : Inport
  Clock : Clock
  Compare To Constant : simulink/Logic and Bit Operations/Compare To Constant  relop=>=  const=max_distance  OutDataTypeStr=boolean
  Constant : Constant  Value=0
  Holding time at the beginning : Subsystem
  Holding time at the end : Subsystem
  Significant speed deviation : Subsystem
  Slope-> angle : Trigonometry  Operator=atan
  Stop Simulation : Stop
  Stop Simulation 2 : Stop
  Switch : Switch  Criteria=u2 > Threshold
  Terminator : Terminator
  altitude : Lookup_n-D  NumberOfTableDimensions=1  BreakpointsForDimension1=cycle.distance  Table=cycle.altitude  InterpMethod=Flat  RndMeth=Simplest  InputSameDT=on
  slope : Lookup_n-D  NumberOfTableDimensions=1  BreakpointsForDimension1=cycle.distance  Table=cycle.slope  InterpMethod=Flat  RndMeth=Simplest  InputSameDT=on
  speed : Lookup_n-D  NumberOfTableDimensions=1  BreakpointsForDimension1=cycle.distance  Table=cycle.speed  InterpMethod=Flat  RndMeth=Simplest  InputSameDT=on
  stop_time : Lookup_n-D  NumberOfTableDimensions=1  BreakpointsForDimension1=cycle.distance  Table=cycle.stop_time  InterpMethod=Flat  RndMeth=Simplest  InputSameDT=on
  v_target [m/s] : Outport
  stop_time [s] : Outport  Port=2
  alpha [rad] : Outport  Port=3
  tag scope: altitude=global, slope_q=global, v_target1=global
  wires:
  slope/1 -> Slope-> angle/1, [slope_q]
  Slope-> angle/1 -> alpha [rad]/1
  Compare To Constant/1 -> Holding time at the end/1(In1)
  Clock/1 -> Terminator/1  "duration"
  Switch/1 -> [v_target1], v_target [m/s]/1
  s_current [m]/1 -> slope/1, Significant speed deviation/1(In1), Compare To Constant/1, altitude/1, speed/1, stop_time/1
  stop_time/1 -> stop_time [s]/1, Switch/2
  speed/1 -> Holding time at the beginning/1(In1)
  Holding time at the end/1(Out1) -> Stop Simulation/1
  Holding time at the beginning/1(Out1) -> Switch/3
  Constant/1 -> Switch/1
  altitude/1 -> [altitude]
  Significant speed deviation/1(Out1) -> Stop Simulation 2/1

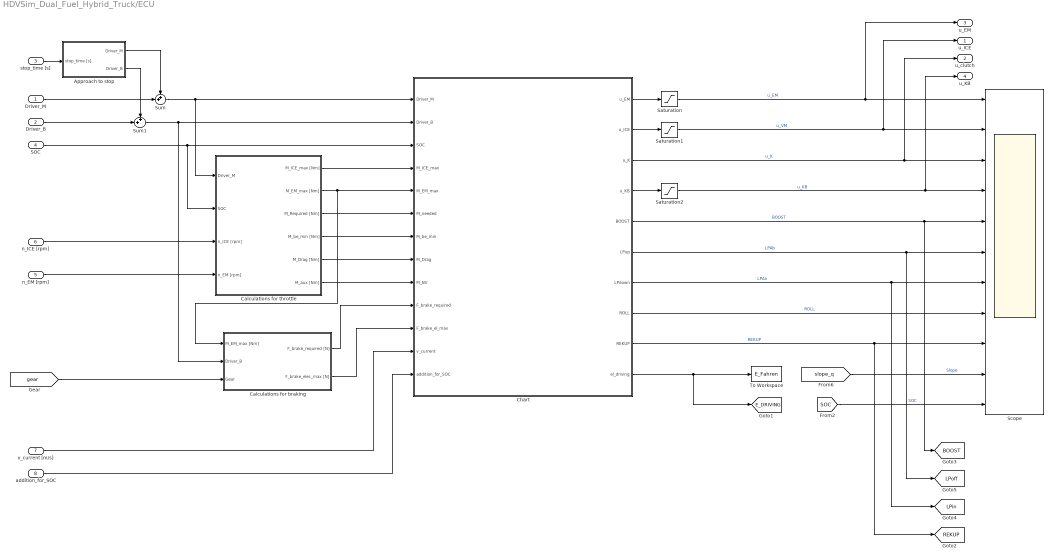
== system HDVSim_Dual_Fuel_Hybrid_Truck/ECU ==
  Driver_M : Inport
  Driver_B : Inport  Port=2
  stop_time [s] : Inport  Port=3
  SOC : Inport  Port=4
  n_EM [rpm] : Inport  Port=5
  n_ICE [rpm] : Inport  Port=6
  v_current [m/s] : Inport  Port=7
  addition_for_SOC : Inport  Port=8
  Approach to stop : Subsystem
  Calculations for braking : Subsystem
  Calculations for throttle : Subsystem
  Chart : Stateflow chart  TreatAsAtomicUnit=on
  Saturation : Saturate  UpperLimit=1  LowerLimit=-1
  Saturation1 : Saturate  UpperLimit=1  LowerLimit=0
  Saturation2 : Saturate  UpperLimit=1  LowerLimit=0
  Scope : Scope  NumInputPorts=11
  Sum : Sum  Inputs=++|
  Sum1 : Sum  Inputs=++|
  To Workspace : ToWorkspace  VariableName=E_Fahren  SampleTime=-1
      settings: Decimation=10
  u_ICE : Outport
  u_clutch : Outport  Port=2
  u_EM : Outport  Port=3
  u_KB : Outport  Port=4
  tag scope: BOOST=global, E_DRIVING=global, LPin=global, LPoff=global, REKUP=global
  wires:
  Chart/1(u_EM) -> Saturation/1
  Chart/2(u_ICE) -> Saturation1/1
  Chart/4(u_KB) -> Saturation2/1
  Sum1/1 -> Calculations for braking/2(Driver_B), Chart/2(Driver_B)
  Sum/1 -> Calculations for throttle/1(Driver_M), Chart/1(Driver_M)
  Chart/3(u_K) -> u_clutch/1, Scope/3  "u_K"
  SOC/1 -> Calculations for throttle/2(SOC), Chart/3(SOC)
  n_ICE [rpm]/1 -> Calculations for throttle/3(n_ICE [rpm])
  Calculations for throttle/1(M_ICE_max [Nm]) -> Chart/4(M_ICE_max)
  Calculations for throttle/3(M_Required [Nm]) -> Chart/6(M_needed)
  Saturation1/1 -> u_ICE/1, Scope/2  "u_VM"
  Saturation2/1 -> u_KB/1, Scope/4  "u_KB"
  Calculations for throttle/5(M_Drag [Nm]) -> Chart/8(M_Drag)
  Calculations for throttle/4(M_be_min [Nm]) -> Chart/7(M_be_min)
  Chart/5(BOOST) -> Scope/5, [BOOST]  "BOOST"
  Chart/8(ROLL) -> Scope/8  "ROLL"
  Chart/9(REKUP) -> [REKUP], Scope/9  "REKUP"
  Chart/7(LPdown) -> [LPin], Scope/7  "LPAn"
  [slope_q] -> Scope/10  "Slope"
  Calculations for throttle/6(M_aux [Nm]) -> Chart/9(M_NV)
  Chart/6(LPup) -> [LPoff], Scope/6  "LPAb"
  Calculations for throttle/2(M_EM_max [Nm]) -> Calculations for braking/1(M_EM_max [Nm]), Chart/5(M_EM_max)
  [SOC] -> Scope/11  "SOC"
  Saturation/1 -> u_EM/1, Scope/1  "u_EM"
  stop_time [s]/1 -> Approach to stop/1(stop_time [s])
  Approach to stop/2(Driver_B) -> Sum1/1
  Approach to stop/1(Driver_M) -> Sum/1
  Driver_M/1 -> Sum/2
  Driver_B/1 -> Sum1/2
  n_EM [rpm]/1 -> Calculations for throttle/4(n_EM [rpm])
  [gear] -> Calculations for braking/3(Gear)
  v_current [m/s]/1 -> Chart/12(v_current)
  Chart/10(el_driving) -> [E_DRIVING], To Workspace/1
  addition_for_SOC/1 -> Chart/13(addition_for_SOC)
  Calculations for braking/1(F_brake_required [N]) -> Chart/10(F_brake_required)
  Calculations for braking/2(F_brake_elec_max [N]) -> Chart/11(F_brake_el_max)

== system HDVSim_Dual_Fuel_Hybrid_Truck/Electric motor ==
  note: Electric torque
  note: Redundant, I_EM_IST is already computed inside the block "Machine current input"
  u_EM : Inport
  n_EM [rpm] : Inport  Port=2
  U_Bat [V] : Inport  Port=3
  Abs : Abs  Commented=on
  Abs1 : Abs
  Divide : Product  Commented=on  Inputs=*/
  Electric machine efficiency mapping : Lookup_n-D  BreakpointsForDimension1=em.efficiency.torque  BreakpointsForDimension2=em.efficiency.speed  Table=em.efficiency.characteristic_map  RndMeth=Simplest  InputSameDT=on
  Electric machine efficiency mapping2 : Lookup_n-D  Commented=on  BreakpointsForDimension1=em.efficiency.torque  BreakpointsForDimension2=em. efficiency.speed  Table=em.efficiency.characteristic_map  RndMeth=Simplest  InputSameDT=on
  Gain : Gain  Commented=on  Gain=2*pi/60
  Machine current demand : Subsystem
  Machine torque demand : Subsystem
  Math Function : Math  Commented=on  Operator=reciprocal  SaturateOnIntegerOverflow=on
  Product1 : Product
  Product2 : Product  Commented=on  Inputs=3
  Saturation : Saturate  UpperLimit=Bat.Useable_capacity / Bat.Useable_range*10  LowerLimit=-Bat.Useable_capacity / Bat.Useable_range*10
  Saturation1 : Saturate  Commented=on  UpperLimit=inf  LowerLimit=1
  Speed-torrque characteristics : Lookup_n-D  NumberOfTableDimensions=1  BreakpointsForDimension1=em.speed  Table=em.trq  ExtrapMethod=Clip  RndMeth=Simplest  InputSameDT=on
  Switch : Switch  Commented=on
  M_EM [Nm] : Outport
  I_EM_current [A] : Outport  Port=2
  tag scope: M_EM=global, n_EM=global, u_EM=global
  wires:
  Speed-torrque characteristics/1 -> Product1/1  "M_EM_max"
  u_EM/1 -> Product1/2, [u_EM]
  U_Bat [V]/1 -> Divide/2, Machine torque demand/4(U_Bat [V]), Machine current demand/4(U_Bat [V])
  Machine current demand/1(I_target [A]) -> Saturation/1
  Machine torque demand/1(M_EM [Nm]) -> Product2/3, [M_EM], M_EM [Nm]/1, Switch/2, Abs/1
  Gain/1 -> Product2/2
  Math Function/1 -> Switch/1
  Electric machine efficiency mapping2/1 -> Switch/3, Math Function/1  "Eta_EM"
  Switch/1 -> Product2/1
  Product2/1 -> Divide/1
  Abs/1 -> Electric machine efficiency mapping2/1
  Product1/1 -> Machine current demand/2(M_EM_target [Nm]), Abs1/1  "M_EM_soll"
  n_EM [rpm]/1 -> Electric machine efficiency mapping/2, Saturation1/1, Electric machine efficiency mapping2/2, Machine torque demand/1(n_EM [rpm]), Machine current demand/1("n_EM "), [n_EM], Speed-torrque characteristics/1
  Abs1/1 -> Electric machine efficiency mapping/1
  Electric machine efficiency mapping/1 -> Machine current demand/3(Eff_EM), Machine torque demand/3(Eff_EM)  "ETA_EM"
  Saturation1/1 -> Gain/1
  Saturation/1 -> Machine torque demand/2(I_current [A]), I_EM_current [A]/1

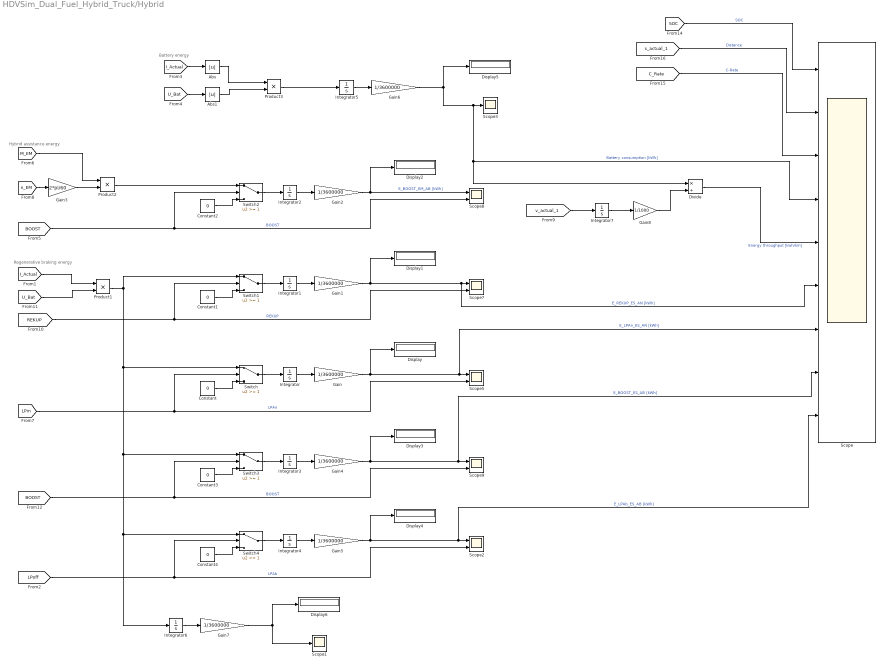
== system HDVSim_Dual_Fuel_Hybrid_Truck/Hybrid ==
  note: Battery energy
  note: Hybrid assistance energy
  note: Regenerative braking energy
  Abs : Abs
  Abs1 : Abs
  Constant{,1..4} (5 alike) : Constant  Value=0
  Display{,1..6} (7 alike) : Display
  Divide : Product  Inputs=*/
  Gain{,1..2,4..7} (7 alike) : Gain  Gain=1/3600000
  Gain3 : Gain  Gain=2*pi/60
  Gain8 : Gain  Gain=1/1000
  Integrator{,1..6} (7 alike) : Integrator
  Integrator7 : Integrator  InitialCondition=0.00000001
  Product1 : Product
  Product2 : Product
  Product3 : Product
  Scope : Scope  NumInputPorts=9
  Scope1 : Scope
  Scope{2,5,7..9} (5 alike) : Scope  NumInputPorts=2
  Scope3 : Scope
  Switch{,1..4} (5 alike) : Switch  Threshold=1
  wires:
  Product1/1 -> Switch1/1, Switch/1, Switch3/1, Integrator6/1, Switch4/1
  Gain5/1 -> Scope/9, Scope2/1, Display4/1  "E_LPAb_ES_AB [kWh]"
  Constant4/1 -> Switch4/3
  Integrator4/1 -> Gain5/1
  Switch4/1 -> Integrator4/1
  [LPoff] -> Scope2/2, Switch4/2  "LPAb"
  Gain4/1 -> Scope/8, Scope9/1, Display3/1  "E_BOOST_ES_AB [kWh]"
  Constant3/1 -> Switch3/3
  Integrator3/1 -> Gain4/1
  Switch3/1 -> Integrator3/1
  [BOOST] -> Scope9/2, Switch3/2  "BOOST"
  Gain3/1 -> Product2/2
  [n_EM] -> Gain3/1
  Gain2/1 -> Scope8/1, Display2/1  "E_BOOST_EM_AB [kWh]"
  Constant2/1 -> Switch2/3
  Integrator2/1 -> Gain2/1
  Switch2/1 -> Integrator2/1
  [BOOST] -> Scope8/2, Switch2/2  "BOOST"
  Product2/1 -> Switch2/1
  Gain1/1 -> Scope/6, Scope7/1, Display1/1  "E_REKUP_ES_AN [kWh]"
  Constant1/1 -> Switch1/3
  Integrator1/1 -> Gain1/1
  Switch1/1 -> Integrator1/1
  [REKUP] -> Scope7/2, Switch1/2  "REKUP"
  [U_Bat] -> Product1/2
  [I_Actual] -> Product1/1
  Gain/1 -> Scope/7, Scope5/1, Display/1  "E_LPAn_ES_AN [kWh]"
  Constant/1 -> Switch/3
  Integrator/1 -> Gain/1
  Switch/1 -> Integrator/1
  [LPin] -> Scope5/2, Switch/2  "LPAn"
  [M_EM] -> Product2/1
  Gain7/1 -> Display6/1, Scope1/1
  Integrator6/1 -> Gain7/1
  [U_Bat] -> Abs1/1
  [I_Actual] -> Abs/1
  Product3/1 -> Integrator5/1
  Integrator5/1 -> Gain6/1
  Abs/1 -> Product3/1
  Abs1/1 -> Product3/2
  [SOC] -> Scope/1  "SOC"
  Gain6/1 -> Display5/1, Scope/4, Divide/1, Scope3/1  "Battery consumption [kWh]"
  [s_actual_1] -> Scope/2  "Distance"
  [C_Rate] -> Scope/3  "C-Rate"
  Divide/1 -> Scope/5  "Energy throughput [kwh/km]"
  [v_actual_1] -> Integrator7/1
  Integrator7/1 -> Gain8/1
  Gain8/1 -> Divide/2

== system HDVSim_Dual_Fuel_Hybrid_Truck/ICE engine ==
  note: Consumption calculations
  note: Engine loading
  u_ICE : Inport
  n_ICE [rpm] : Inport  Port=2
  Additional consumptions : Subsystem
  Consumption : Subsystem
  Drag torque : Lookup  InputValues=engine.drag_torque.speed  Table=engine.drag_torque.trq  LookUpMeth=Interpolation-Use End Values
  Full load curve : Lookup  InputValues=engine.full_load.speed  Table=engine.full_load.trq  LookUpMeth=Interpolation-Use End Values
  MinMax : MinMax  Inputs=2
  Product1 : Product
  Sum : Sum  Inputs=|+-
  Sum1 : Sum  Inputs=|++
  maximum engine torque due to tire slip : Subsystem
  M_ICE [Nm] : Outport
  tag scope: M_mot=global, n_mot=global
  wires:
  n_ICE [rpm]/1 -> Consumption/2(n [rpm]), Additional consumptions/2(n_clutch_en [rpm]), [n_mot], Drag torque/1, Full load curve/1
  Sum/1 -> Product1/2
  Product1/1 -> Sum1/1
  Drag torque/1 -> Sum1/2, Sum/2  "M_Drag"
  Additional consumptions/1(M_ICE_aftr_aux [Nm]) -> M_ICE [Nm]/1
  u_ICE/1 -> Product1/1
  Full load curve/1 -> MinMax/2  "M_VM_max"
  Sum1/1 -> Consumption/1(M [Nm]), [M_mot], Additional consumptions/1(M_ICE_bfor_aux [Nm])
  maximum engine torque due to tire slip/1(M_mot_max_traction [Nm]) -> MinMax/1
  MinMax/1 -> Sum/1

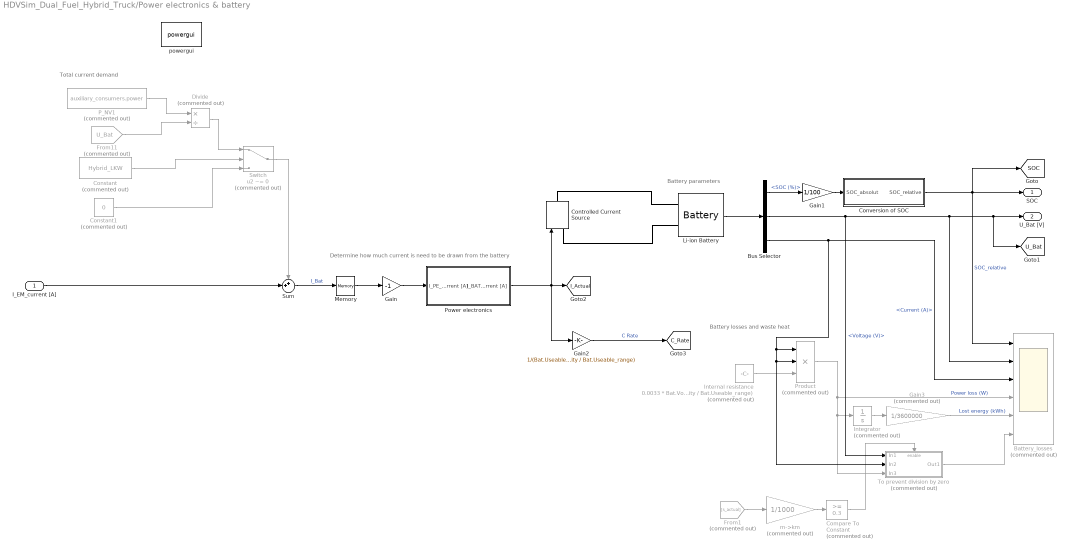
== system HDVSim_Dual_Fuel_Hybrid_Truck/Power electronics & battery ==
  note: Battery parameters
  note: Determine how much current is need to be drawn from the battery
  note: Total current demand
  note: Battery losses and waste heat
  I_EM_current [A] : Inport
  Battery_losses : Scope  Commented=on  NumInputPorts=6
  Bus Selector : BusSelector  OutputSignals=SOC (%),Voltage (V),Current (A)
  Compare To Constant : simulink/Logic and Bit Operations/Compare To Constant  Commented=on  relop=>=  const=0.3  OutDataTypeStr=uint8  ZeroCross=off
  Constant : Constant  Commented=on  Value=Hybrid_LKW
  Constant1 : Constant  Commented=on  Value=0
  Controlled Current Source : powerlib/Electrical Sources/Controlled Current Source  Initialize=off  Source_Type=DC  Amplitude=0  Phase=0  Frequency=0  Measurements=None
      settings: SourceProductName=Simscape Electrical
  Conversion of SOC : Subsystem
  Divide : Product  Commented=on  Inputs=*/
  From1 : From  Commented=on  GotoTag=s_actual  TagVisibility=global
      settings: CloseFcn=tagdialog Close
  From11 : From  Commented=on  GotoTag=U_Bat  TagVisibility=global
  Gain : Gain  Gain=-1
  Gain1 : Gain  Gain=1/100
  Gain2 : Gain  Gain=1/(Bat.Useable_capacity / Bat.Useable_range)
  Gain3 : Gain  Commented=on  Gain=1/3600000
  Integrator : Integrator  Commented=on
  Internal resistance : Constant  Commented=on  Value=0.0033 * Bat.Voltage / (Bat.Useable_capacity / Bat.Useable_range)
  Li-ion Battery : electricdrivelib/Extra Sources/Battery  BatType=Lithium-Ion  ShowTempParam=off  ThermalPreset=no  ShowAgeParam=off  NomV=Bat.Voltage  NomQ=Bat.Useable_capacity / Bat.Useable_range  SOC=(Bat.SOC_start *Bat.Useable_range+(0.5-Bat.Useable_range/2))* 100  Batt_Tr=30  PresetModel=off  MaxQ=Bat.Useable_capacity / Bat.Useable_range *8077/7500  MinV=487.5  FullV=Bat.Voltage * 1.178  Dis_rate=Bat.Useable_capacity / Bat.Useable_range * 1  R=0.0033 * Bat.Voltage / (Bat.Useable_capacity / Bat.Useable_range)  Normal_OP=Bat.Useable_capacity / Bat.Useable_range * 0.962  expZone="[Bat.Voltage*4339/4000     Bat.Useable_capacity / Bat.Useable_range/5]"  current=[5 25 50 250]  Units=Ampere-hour  Tci=20  NomT=20  T2=-30  MaxQ2=4.8  FullV2=7.1  Normal_OP2=5.72  expZone2="[6.58  1]"  Rca=0.6  ti=1000  Dp=0  Neq0=0  Tsim=1e6  Ta1=25  Qeol=5.4*0.9  Reol=0.013333*1.2  Char_age=[2.3478, 3]  Dis_age=[2.3478, 10]  N1=1500  N2=10500  N3=1000  N4=1400  Ta2=45  N5=950
      settings: SourceProductName=Simscape Electrical
  Memory : Memory
  P_NV1 : Constant  Commented=on  Value=auxiliary_consumers.power
  Power electronics : Subsystem
  Product : Product  Commented=on  Inputs=3
  Sum : Sum  Inputs=++|
  Switch : Switch  Commented=on  Criteria=u2 ~= 0
  To prevent division by zero : Subsystem  Commented=on
  m->km : Gain  Commented=on  Gain=1/1000
  powergui : powerlib/powergui  Priority=1  SimulationMode=Discrete  SampleTime=sample_time  frequency=60  Iterations=50  frequencyindice=0  Pbase=100e6  ErrMax=1e-4  UnitsV=kV  UnitsW=MW  buscounter=0  FunctionMessages=off  echomessages=off  EnableUseOfTLC=off  CurrentSourceSwitches=off  DisableSnubberDevices=off  DisableRonSwitches=off  DisableVfSwitches=off  DisplayEquations=off  SolverType=Tustin  Interpol=off  ExternalGateDelay=off  methode=off  Ts=100  x0status=blocks  SPID=off  SwTol=0  HookPort=off  RestoreLinks=warning  ResistiveCurrentMeasurement=off  Frange=[0:2:500]  Ylog=off  Xlog=on  ShowGrid=off  save=off  variable=ZData  structure=0  ZoomFFT=off  StartTime=0.0  cycles=1  DisplayStyle=1  fundamental=60  FreqAxis=off  MaxFrequency=1000  frequencyindicesteady=1  RmsSteady=1  display=off
  SOC : Outport
  U_Bat [V] : Outport  Port=2
  tag scope: C_Rate=global, I_Actual=global, SOC=global, U_Bat=global
  wires:
  Li-ion Battery/1 -> Bus Selector/1
  Bus Selector/1 -> Gain1/1  "<SOC (%)>"
  Gain1/1 -> Conversion of SOC/1(SOC_absolut)
  Conversion of SOC/1(SOC_relative) -> SOC/1, [SOC], Battery_losses/1  "SOC_relative"
  Memory/1 -> Gain/1
  Gain/1 -> Power electronics/1(I_PE_current [A])
  Power electronics/1(I_BAT_current [A]) -> Gain2/1, Controlled Current Source/1, [I_Actual]
  Gain2/1 -> [C_Rate]  "C Rate"
  From11/1 -> Divide/2
  Sum/1 -> Memory/1  "I_Bat"
  Constant1/1 -> Switch/3
  P_NV1/1 -> Divide/1
  Divide/1 -> Switch/1
  I_EM_current [A]/1 -> Sum/2
  Switch/1 -> Sum/1
  Constant/1 -> Switch/2
  m->km/1 -> Compare To Constant/1
  Compare To Constant/1 -> To prevent division by zero/Enable
  From1/1 -> m->km/1
  Gain3/1 -> Battery_losses/5  "Lost energy (kWh)"
  To prevent division by zero/1(Out1) -> Battery_losses/6
  Internal resistance/1 -> Product/3
  Integrator/1 -> Gain3/1
  Product/1 -> Battery_losses/4, To prevent division by zero/3(In3), Integrator/1  "Power loss (W)"
  Bus Selector/3 -> Product/1, Product/2, To prevent division by zero/2(In2), Battery_losses/3  "<Current (A)>"
  Bus Selector/2 -> To prevent division by zero/1(In1), Battery_losses/2, [U_Bat], U_Bat [V]/1  "<Voltage (V)>"
  connections:
  Li-ion Battery/LConn1 -- Controlled Current Source/RConn1
  Li-ion Battery/LConn2 -- Controlled Current Source/LConn1

== system HDVSim_Dual_Fuel_Hybrid_Truck/Tires ==
  M_tire [Nm] : Inport
  v_current [m/s] : Inport  Port=2
  F=M/r : Product  Inputs=*/
  Tire radius : Constant  Value=tires.radius
  "phi. -> n[1/min]" : Gain  Gain=60/2/pi
  phi. = v/r : Product  Inputs=/*
  n_tire [rpm] : Outport
  F_x [N] : Outport  Port=2
  wires:
  phi. = v/r/1 -> "phi. -> n[1/min]"/1
  "phi. -> n[1/min]"/1 -> n_tire [rpm]/1
  Tire radius/1 -> phi. = v/r/1, F=M/r/2
  v_current [m/s]/1 -> phi. = v/r/2
  M_tire [Nm]/1 -> F=M/r/1
  F=M/r/1 -> F_x [N]/1

== system HDVSim_Dual_Fuel_Hybrid_Truck/Transmission ==
  note: Transmission torque multiplication through the different gears
  M_EM [Nm] : Inport
  M_clutch_dis [Nm] : Inport  Port=2
  n_Gearbox [rpm] : Inport  Port=3
  alpha : Inport  Port=4
  Determine when shifting occurs : Subsystem  TreatAsAtomicUnit=on
  Memory1 : Memory
  Number of gears : Constant  Value=length(transmission.ratios)
  Saturation : Saturate  UpperLimit=2000  LowerLimit=0
  Shifting strategy : Stateflow chart  TreatAsAtomicUnit=on
  Sum : Sum
  Torque flow through the transmission : Subsystem
  ZKU : Subsystem
  init_gear : Constant  Value=transmission.init_gear
  n_clutch_dis [rpm] : Outport
  M_Gearbox [Nm] : Outport  Port=2
  tag scope: gear=global, i_gearbox=global, recommend_DOWN_now=global, recommend_UP_now=global
  wires:
  n_Gearbox [rpm]/1 -> Torque flow through the transmission/2(n_gearbox_out [1/min]), Determine when shifting occurs/2(n_Getr_out [1/min])
  Torque flow through the transmission/2(M_gearbox_out [Nm]) -> [M_gear_ex], M_Gearbox [Nm]/1
  Torque flow through the transmission/1(n_gearbox_in [1/min]) -> Saturation/1
  init_gear/1 -> Shifting strategy/1(init_gear)
  Determine when shifting occurs/27(check_torque_reseve_2lower) -> Shifting strategy/29(check_torque_reserve_2lower)
  Determine when shifting occurs/26(check_torque_reseve_2higher) -> Shifting strategy/28(check_torque_reserve_2higher)
  Determine when shifting occurs/1(reccommend_down_2higher) -> Shifting strategy/3(recommend_down_2higher)
  Determine when shifting occurs/2(reccommend_down_1higher) -> Shifting strategy/4(recommend_down_1higher)
  Determine when shifting occurs/3(reccommend_down_now) -> Shifting strategy/5(recommend_down_now), [recommend_DOWN_now]
  Determine when shifting occurs/4(reccommend_down_1lower) -> Shifting strategy/6(recommend_down_1lower)
  Determine when shifting occurs/5(reccommend_down_2lower) -> Shifting strategy/7(recommend_down_2llower)
  Determine when shifting occurs/6(reccommend_up_2higher) -> Shifting strategy/8(recommend_up_2higher)
  Determine when shifting occurs/7(reccommend_up_1higher) -> Shifting strategy/9(recommend_up_1higher)
  Determine when shifting occurs/8(reccommend_up_now) -> Shifting strategy/10(recommend_up_now), [recommend_UP_now]
  Determine when shifting occurs/9(reccommend_up_1lower) -> Shifting strategy/11(recommend_up_1lower)
  Determine when shifting occurs/10(reccommend_up_2lower) -> Shifting strategy/12(recommend_up_2lower)
  Determine when shifting occurs/11(check_n_min_2higher) -> Shifting strategy/13(check_n_min_2higher)
  Determine when shifting occurs/12(check_n_min_1higher) -> Shifting strategy/14(check_n_min_1higher)
  Determine when shifting occurs/13(check_n_min_now) -> Shifting strategy/15(check_n_min_now)
  Determine when shifting occurs/14(check_n_min_1lower) -> Shifting strategy/16(check_n_min_1lower)
  Determine when shifting occurs/15(check_n_min_2lower) -> Shifting strategy/17(check_n_min_2lower)
  Determine when shifting occurs/16(check_n_max_2higher) -> Shifting strategy/18(check_n_max_2higher)
  Determine when shifting occurs/17(check_n_max_1higher) -> Shifting strategy/19(check_n_max_1higher)
  Determine when shifting occurs/18(check_n_max_now) -> Shifting strategy/20(check_n_max_now)
  Determine when shifting occurs/19(check_n_max_1lower) -> Shifting strategy/21(check_n_max_1lower)
  Determine when shifting occurs/20(check_n_max_2lower) -> Shifting strategy/22(check_n_max_2lower)
  Determine when shifting occurs/21(check_M_max_2higher) -> Shifting strategy/23(check_M_max_2higher)  "check_M_max_2higher"
  Determine when shifting occurs/22(check_M_max_1higher) -> Shifting strategy/24(check_M_max_1higher)  "check_M_max_1higher"
  Determine when shifting occurs/23(check_M_max_now) -> Shifting strategy/25(check_M_max_now)  "check_M_max_now"
  Determine when shifting occurs/24(check_M_max_1lower) -> Shifting strategy/26(check_M_max_1lower)  "check_M_max_1lower"
  Determine when shifting occurs/25(check_M_max_2lower) -> Shifting strategy/27(check_M_max_2lower)  "check_M_max_2lower"
  Memory1/1 -> [Gear], ZKU/1(Gear), Torque flow through the transmission/3(Gear), [gear]
  M_clutch_dis [Nm]/1 -> Sum/2
  Sum/1 -> Torque flow through the transmission/1(M_gearbox_in [Nm])  "M_gearbox_in [Nm]"
  Torque flow through the transmission/3(i_gearbox) -> [i_gearbox]
  Saturation/1 -> n_clutch_dis [rpm]/1
  M_EM [Nm]/1 -> Sum/1, Determine when shifting occurs/4(M_EM [Nm])
  Number of gears/1 -> Shifting strategy/2(z)
  alpha/1 -> Determine when shifting occurs/5(alpha)
  Shifting strategy/1(gear) -> [gear]
  [gear] -> Memory1/1
  [Gear] -> Determine when shifting occurs/1(Gear)
  [M_gear_ex] -> Determine when shifting occurs/3(M_Getr_out [Nm])

== system HDVSim_Dual_Fuel_Hybrid_Truck/Vehicle ==
  note: Vehicle acceleration
  note: Net tractive force applied on the vehicle
  F_x [N] : Inport
  u_KB : Inport  Port=2
  alpha [rad] : Inport  Port=3
  Add : Sum  Inputs=-+-
  Braking force [N] : Product  RndMeth=Zero
  Cargo weight : Constant  Value=vehicle.payload
  Driving resistances without acceleration : Subsystem
  F_brake_max : Constant  Value=vehicle.F_brake_max
  Integrator : Integrator
  Integrator1 : Integrator  InitialCondition=cycle.speed_init  LimitOutput=on  LowerSaturationLimit=0
  Product2 : Product  Inputs=*/  RndMeth=Zero
  Product3 : Product  Inputs=**  RndMeth=Zero
  Saturation : Saturate  UpperLimit=15  LowerLimit=-15
  Sum1 : Sum  Inputs=|++
  Vehicle weight : Constant  Value=vehicle.mass
  v_current [m/s] : Outport
  s_current [m] : Outport  Port=2
  tag scope: s_actual_1=global, v_actual_1=global
  wires:
  alpha [rad]/1 -> Driving resistances without acceleration/1(alpha [rad])
  Add/1 -> Product2/1
  Driving resistances without acceleration/1(F_W [N]) -> Add/3
  F_x [N]/1 -> Add/2  "F_x"
  F_brake_max/1 -> Braking force [N]/2
  Integrator/1 -> [s_actual_1], s_current [m]/1  "s_ist"
  Cargo weight/1 -> Sum1/2
  Sum1/1 -> Product2/2
  Vehicle weight/1 -> Product3/2
  Product3/1 -> Sum1/1
  Integrator1/1 -> Integrator/1, Driving resistances without acceleration/2(v [m/s]), v_current [m/s]/1, [v_actual_1]  "v_ist"
  [lamda] -> Product3/1
  u_KB/1 -> Braking force [N]/1
  Braking force [N]/1 -> Add/1  "F_Brake"
  Product2/1 -> Saturation/1  "a"
  Saturation/1 -> Integrator1/1

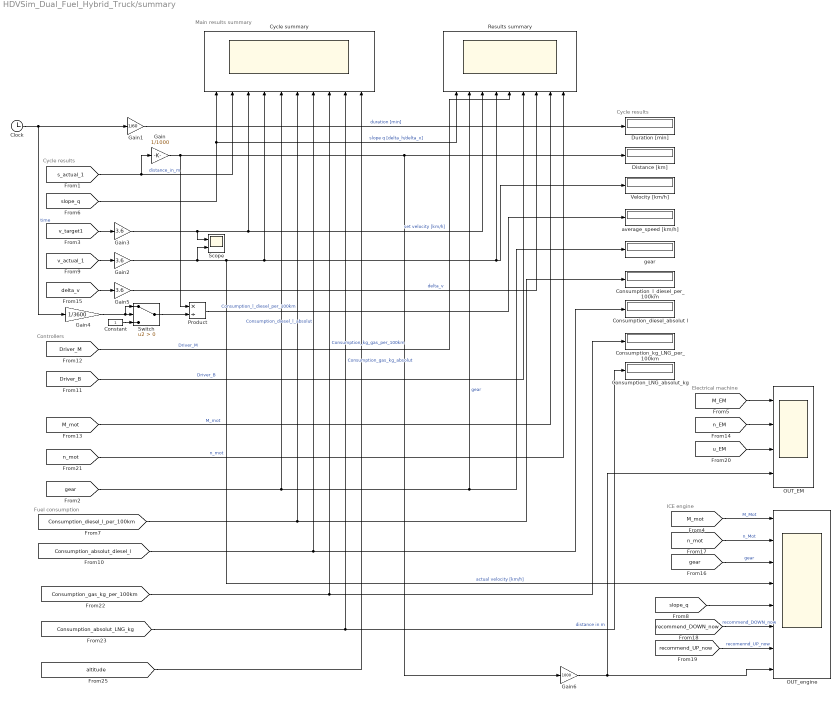
== system HDVSim_Dual_Fuel_Hybrid_Truck/summary ==
  note: Cycle results
  note: Electrical machine
  note: ICE engine
  note: Fuel consumption
  note: Controllers
  note: Cycle results
  note: Main results summary
  Clock : Clock
  Constant : Constant
  Consumption_LNG_absolut_kg : Display
  Consumption_diesel_absolut l : Display
  Consumption_kg_LNG_per_100km : Display
  Consumption_l_diesel_per_100km : Display
  Cycle summary : Scope  NumInputPorts=10
  Distance [km] : Display
  Duration [min] : Display
  Gain : Gain  Gain=1/1000
  Gain1 : Gain  Gain=1/60
  Gain2 : Gain  Gain=3.6
  Gain3 : Gain  Gain=3.6
  Gain4 : Gain  Gain=1/3600
  Gain5 : Gain  Gain=3.6
  Gain6 : Gain  Gain=1000
  OUT_EM : Scope  NumInputPorts=4
  OUT_engine : Scope  NumInputPorts=8
  Product : Product  Inputs=*/  RndMeth=Zero
  Results summary : Scope  NumInputPorts=9
  Scope : Scope  NumInputPorts=2
  Switch : Switch  Criteria=u2 > Threshold
  Velocity [km/h] : Display
  average_speed [km/h] : Display
  gear : Display
  wires:
  [v_actual_1] -> Gain2/1
  [s_actual_1] -> Cycle summary/2, Gain/1  "distance_in_m"
  Gain/1 -> Gain6/1, Distance [km]/1, Product/1
  Clock/1 -> Gain1/1, Gain4/1  "time"
  Gain1/1 -> Duration [min]/1  "duration [min]"
  Gain2/1 -> Scope/2, Results summary/4, Velocity [km/h]/1, Cycle summary/4, OUT_engine/4  "actual velocity [km/h]"
  [gear] -> Results summary/2, gear/1, Cycle summary/5  "gear"
  [v_target1] -> Gain3/1
  [slope_q] -> Results summary/1, Cycle summary/1  "slope q [delta_h/delta_x]"
  [Consumption_diesel_l_per_100km] -> Consumption_l_diesel_per_100km/1, Cycle summary/6  "Consumption_l_diesel_per_100km"
  Gain3/1 -> Scope/1, Results summary/3, Cycle summary/3  "set velocity [km/h]"
  Gain4/1 -> Switch/1, Switch/2
  Product/1 -> average_speed [km/h]/1
  [Consumption_absolut_diesel_l] -> Consumption_diesel_absolut l/1, Cycle summary/7  "Consumption_diesel_l_absolut"
  [Driver_M] -> Results summary/5  "Driver_M"
  [Driver_B] -> Results summary/6  "Driver_B"
  [M_mot] -> Results summary/8  "M_mot"
  [delta_v] -> Gain5/1
  [M_mot] -> OUT_engine/1  "M_Mot"
  [n_mot] -> OUT_engine/2  "n_Mot"
  [gear] -> OUT_engine/3  "gear"
  [recommend_DOWN_now] -> OUT_engine/6  "recommend_DOWN_now"
  [recommend_UP_now] -> OUT_engine/7  "recomennd_UP_now"
  [slope_q] -> OUT_engine/5
  Gain5/1 -> Results summary/7  "delta_v"
  [n_mot] -> Results summary/9  "n_mot"
  [M_EM] -> OUT_EM/1
  [n_EM] -> OUT_EM/2
  [u_EM] -> OUT_EM/3
  [Consumption_gas_kg_per_100km] -> Cycle summary/8, Consumption_kg_LNG_per_100km/1  "Consumption_kg_gas_per_100km"
  [Consumption_absolut_LNG_kg] -> Consumption_LNG_absolut_kg/1, Cycle summary/9  "Consumption_gas_kg_absolut"
  Switch/1 -> Product/2
  Constant/1 -> Switch/3
  [altitude] -> Cycle summary/10
  Gain6/1 -> OUT_EM/4, OUT_engine/8  "distance in m"

== system HDVSim_Dual_Fuel_Hybrid_Truck/Active cruise control/Braking from upper speed limit ==
  v_target [m/s] : Inport
  Add3 : Sum  Inputs=+-
  Constant1 : Constant  Value=90/3.6
  Constant10 : Constant  Value=preditiveCruiseControl
  Constant6 : Constant  Value=v_PPC_delta
  Constant7 : Constant  Value=0
  Constant8 : Constant  Value=0
  Saturation Dynamic : simulink/Discontinuities/Saturation Dynamic  OutMin=[]  OutMax=[]  OutDataTypeStr=Inherit: Same as second input  OutDataType=fixdt(1, 16)  OutScaling=2^-10  DoSatur=off
  Switch3 : Switch  Criteria=u2 > Threshold
  Out1 : Outport
  wires:
  Switch3/1 -> Out1/1
  Constant6/1 -> Saturation Dynamic/2
  Constant1/1 -> Add3/1
  Constant7/1 -> Switch3/3
  Add3/1 -> Saturation Dynamic/1
  Constant8/1 -> Saturation Dynamic/3
  Constant10/1 -> Switch3/2
  v_target [m/s]/1 -> Add3/2
  Saturation Dynamic/1 -> Switch3/1
